simulink model "controller"  (Simulink 8.8)
settings: Solver=VariableStepAuto  StartTime=0.0  StopTime=10.0  RelTol=1e-3
undefined symbols (not defined in the file): L, R, Ta, Td
settings Model: Creator=KGOSWAM  LastModifiedBy=KGOSWAM
settings DataIOCC: LimitDataPoints=off  SaveFormat=Dataset  SignalLoggingSaveFormat=Dataset
settings OptimizationCC: LifeSpan=auto
settings DebuggingCC: UnderspecifiedInitializationDetection=Simplified  MergeDetectMultiDrivingBlocksExec=error  FcnCallInpInsideContextMsg=error  StateNameClashWarn=none  SFUnexpectedBacktrackingDiag=error  SFNoUnconditionalDefaultTransitionDiag=error  SFExecutionAtInitializationDiag=warning
settings HardwareCC: ProdBitPerPointer=64  ProdBitPerSizeT=64  ProdBitPerPtrDiffT=64  ProdLargestAtomicFloat=Float  ProdIntDivRoundTo=Zero  ProdEndianess=LittleEndian  ProdWordSize=64  ProdHWDeviceType=Intel->x86-64 (Windows64)
settings ModelReferenceCC: PropagateSignalLabelsOutOfModel=on
settings GRTTargetCC: TargetLangStandard=C99 (ISO)  GeneratePreprocessorConditionals=Use local settings  CombineOutputUpdateFcns=on  GRTInterface=off
settings ConfigComp: CovMetricSettings=dwe  CovHtmlReporting=off  CovSaveCumulativeToWorkspaceVar=off  CovSaveSingleToWorkspaceVar=off  CovExternalEMLEnable=on

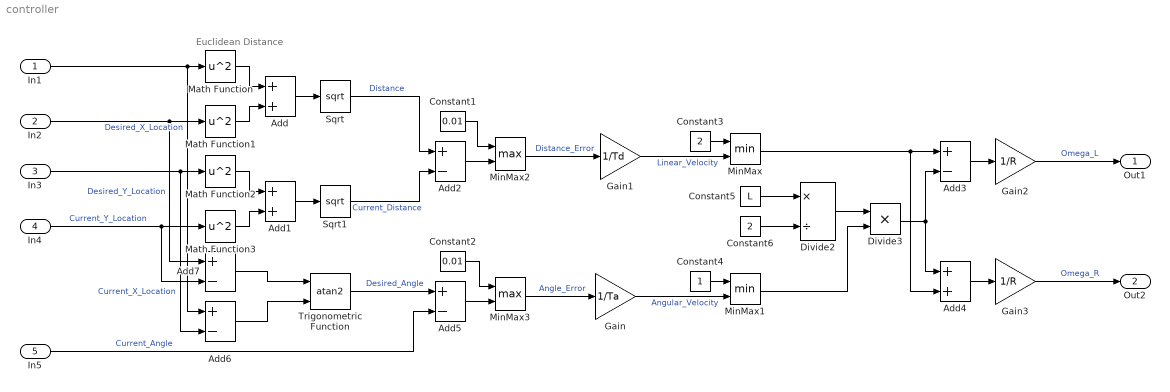
== system controller ==
  note: Euclidean Distance
  In1 : Inport
  In2 : Inport  Port=2
  In3 : Inport  Port=3
  In4 : Inport  Port=4
  In5 : Inport  Port=5
  Add : Sum
  Add1 : Sum
  Add{2..3,5..7} (5 alike) : Sum  Inputs=+-
  Add4 : Sum
  Constant1 : Constant  Value=0.01
  Constant2 : Constant  Value=0.01
  Constant3 : Constant  Value=2
  Constant4 : Constant
  Constant5 : Constant  Value=L
  Constant6 : Constant  Value=2
  Divide2 : Product  Inputs=*/
  Divide3 : Product  Inputs=**
  Gain : Gain  Gain=1/Ta
  Gain1 : Gain  Gain=1/Td
  Gain2 : Gain  Gain=1/R
  Gain3 : Gain  Gain=1/R
  Math Function{,1..3} (4 alike) : Math  Operator=square  SaturateOnIntegerOverflow=on
  MinMax : MinMax  Inputs=2
  MinMax1 : MinMax  Inputs=2
  MinMax2 : MinMax  Function=max  Inputs=2
  MinMax3 : MinMax  Function=max  Inputs=2
  Sqrt : Sqrt  SaturateOnIntegerOverflow=on
  Sqrt1 : Sqrt  SaturateOnIntegerOverflow=on
  Trigonometric Function : Trigonometry  Operator=atan2
  Out1 : Outport
  Out2 : Outport  Port=2
  wires:
  In1/1 -> Add6/1, Math Function/1  "Desired_X_Location"
  In2/1 -> Add7/1, Math Function1/1  "Desired_Y_Location"
  Math Function/1 -> Add/1
  Math Function1/1 -> Add/2
  Add/1 -> Sqrt/1
  Sqrt/1 -> Add2/1  "Distance"
  In3/1 -> Add6/2, Math Function2/1  "Current_X_Location"
  In4/1 -> Add7/2, Math Function3/1  "Current_Y_Location"
  Math Function2/1 -> Add1/1
  Math Function3/1 -> Add1/2
  Add1/1 -> Sqrt1/1
  Sqrt1/1 -> Add2/2  "Current_Distance"
  MinMax2/1 -> Gain1/1  "Distance_Error"
  MinMax3/1 -> Gain/1  "Angle_Error"
  Gain1/1 -> MinMax/2  "Linear_Velocity"
  Constant3/1 -> MinMax/1
  Gain/1 -> MinMax1/2  "Angular_Velocity"
  Constant4/1 -> MinMax1/1
  MinMax/1 -> Add4/2, Add3/1
  Constant5/1 -> Divide2/1
  Constant6/1 -> Divide2/2
  Divide2/1 -> Divide3/1
  MinMax1/1 -> Divide3/2
  Divide3/1 -> Add4/1, Add3/2
  Gain2/1 -> Out1/1  "Omega_L"
  Gain3/1 -> Out2/1  "Omega_R"
  Add7/1 -> Trigonometric Function/1
  Add6/1 -> Trigonometric Function/2
  Trigonometric Function/1 -> Add5/1  "Desired_Angle"
  In5/1 -> Add5/2  "Current_Angle"
  Add2/1 -> MinMax2/2
  Constant1/1 -> MinMax2/1
  Add5/1 -> MinMax3/2
  Constant2/1 -> MinMax3/1
  Add3/1 -> Gain2/1
  Add4/1 -> Gain3/1
